simulink model "ModeloEstimacion"  (R2021a)
settings: Solver=ode4  StartTime=0.0  StopTime=10  FixedStep=0.005  MaxStep=1e-5  MinStep=1e-12  RelTol=1e-3
values from neighbouring files (symbols this model uses):
  A = theta(:,1:end-1)    [EstimacionLeon.m]
  B = (theta(:,end))    [EstimacionLeon.m]
undefined symbols (not defined in the file or in its folder): sigbuilder_block
settings Model: Creator=unam-  LastModifiedBy=jalej
settings DebuggingCC: UnconnectedInputMsg=none  UnconnectedOutputMsg=none  UnconnectedLineMsg=none
settings ModelReferenceCC: EnableRefExpFcnMdlSchedulingChecks=off
settings RTWCC: Description=Generic Real-Time Target  DLArmComputeVersion=20.02.1

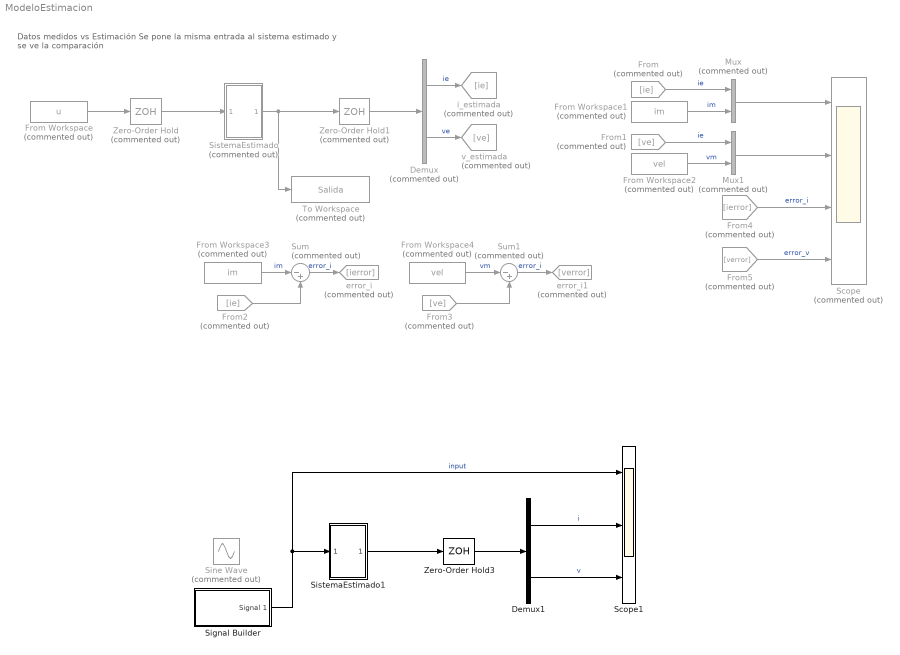
== system ModeloEstimacion ==
  note: Datos medidos vs Estimación
      | Se pone la misma entrada al sistema estimado y se ve la comparación
  Demux : Demux  Commented=on  Outputs=2
  Demux1 : Demux  Outputs=2
  From : From  Commented=on  GotoTag=ie
  From Workspace : FromWorkspace  Commented=on  VariableName=u  SampleTime=0.005
  From Workspace1 : FromWorkspace  Commented=on  VariableName=im
  From Workspace2 : FromWorkspace  Commented=on  VariableName=vel
  From Workspace3 : FromWorkspace  Commented=on  VariableName=im
  From Workspace4 : FromWorkspace  Commented=on  VariableName=vel
  From1 : From  Commented=on  GotoTag=ve
  From2 : From  Commented=on  GotoTag=ie
  From3 : From  Commented=on  GotoTag=ve
  From4 : From  Commented=on  GotoTag=ierror
  From5 : From  Commented=on  GotoTag=verror
  Mux : Mux  Commented=on  Inputs=2
  Mux1 : Mux  Commented=on  Inputs=2
  Scope : Scope  Commented=on  NumInputPorts=4
  Scope1 : Scope  NumInputPorts=3
  Signal Builder : Subsystem  Tag=STV Subsys  LoadFcn=sigbuilder_block('load');  StartFcn=sigbuilder_block('start');  StopFcn=sigbuilder_block('stop');  ClipboardFcn=sigbuilder_block('clipboard');  mask(Sigbuilder block){tuvar=[0:10]}
      mask help: Simulink:masks:SigbuilderBlock_MD
      mask init:
      | if ~strcmp(get_param(bdroot(gcbh),'SimulationStatus'),'stopped') tuvar = sigbuilder_block('maskInit'); end
      settings: CopyFcn=sigbuilder_block('copy');  DeleteFcn=sigbuilder_block('delete');  ModelCloseFcn=sigbuilder_block('modelClose');  PreSaveFcn=sigbuilder_block('preSave');  PauseFcn=sigbuilder_block('pause');  ContinueFcn=sigbuilder_block('continue');  NameChangeFcn=sigbuilder_block('namechange');  OpenFcn=sigbuilder_block('open',[437.6 199.2 550.4 400 ]);  CloseFcn=sigbuilder_block('close');
      mask Display: plot(0, 0, 100, 100,[2, 2, 32, 32, 2], [68, 8, 8, 68, 68],[32, 2], [38, 38], [32, 19, 2],[53, 60, 44], [32, 17, 17, 2],[16, 16, 31, 31]);txt = getActiveGroup(gcbh);text(2, 100, txt,'verticalAlignment', 'top');
  Sine Wave : Sin  Commented=on  Amplitude=6  Bias=6  SampleTime=0.005
  SistemaEstimado : Subsystem  Commented=on
  SistemaEstimado1 : Subsystem
  Sum : Sum  Commented=on  Inputs=|-+
  Sum1 : Sum  Commented=on  Inputs=|-+
  To Workspace : ToWorkspace  Commented=on  VariableName=Salida  SaveFormat=Timeseries  SampleTime=0.005
  Zero-Order Hold : ZeroOrderHold  Commented=on  SampleTime=0.005
  Zero-Order Hold1 : ZeroOrderHold  Commented=on  SampleTime=0.005
  Zero-Order Hold3 : ZeroOrderHold  SampleTime=0.005
  error_i : Goto  Commented=on  GotoTag=ierror
  error_i1 : Goto  Commented=on  GotoTag=verror
  i_estimada : Goto  Commented=on  GotoTag=ie
  v_estimada : Goto  Commented=on  GotoTag=ve
  wires:
  SistemaEstimado/1(Out1) -> To Workspace/1, Zero-Order Hold1/1
  Zero-Order Hold/1 -> SistemaEstimado/1(In1)
  Zero-Order Hold1/1 -> Demux/1
  From Workspace/1 -> Zero-Order Hold/1
  From Workspace2/1 -> Mux1/2  "vm"
  From Workspace1/1 -> Mux/2  "im"
  Mux/1 -> Scope/1
  Mux1/1 -> Scope/2
  Demux/1 -> i_estimada/1  "ie"
  Demux/2 -> v_estimada/1  "ve"
  From/1 -> Mux/1  "ie"
  From1/1 -> Mux1/1  "ie"
  From Workspace3/1 -> Sum/1  "im"
  From2/1 -> Sum/2
  Sum/1 -> error_i/1  "error_i"
  From Workspace4/1 -> Sum1/1  "vm"
  From3/1 -> Sum1/2
  Sum1/1 -> error_i1/1  "error_i"
  From4/1 -> Scope/3  "error_i"
  From5/1 -> Scope/4  "error_v"
  Demux1/2 -> Scope1/3  "v"
  SistemaEstimado1/1(Out1) -> Zero-Order Hold3/1
  Demux1/1 -> Scope1/2  "i"
  Zero-Order Hold3/1 -> Demux1/1
  Signal Builder/1(Signal 1) -> Scope1/1, SistemaEstimado1/1(In1)  "input"

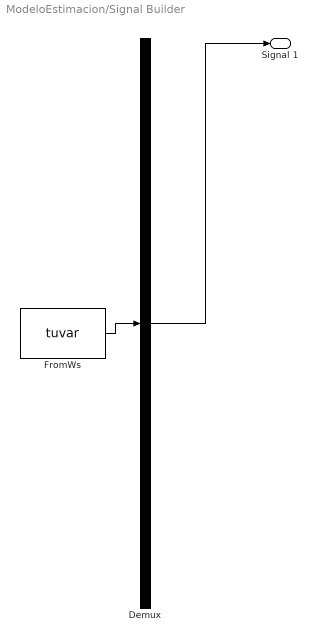
== system ModeloEstimacion/Signal Builder ==
  Demux : Demux  Tag=STV Demux  Outputs=1
      settings: DisplayOption=none
  FromWs : FromWorkspace  Tag=STV FromWs  VariableName=tuvar  SampleTime=0.005
      SigBuilderData=|
      | common.afterFinalStr = 'Extrapolate'
      | common.sampleTime = '0.005'
      | dataSet.timeRange = [0 10]
      | dataSet.name = 'Group 1'
      | sbobj.Groups.Name = 'Group 1'
      | sbobj.Groups.Signals.Name = 'Signal 1'
      | sbobj.Groups.Signals.XData = [0 2 2 9.02 9.02 10]
      | sbobj.Groups.Signals.YData = [0 0 12 12 0 0]
  Signal 1 : Outport  Tag=STV Outport
  wires:
  Demux/1 -> Signal 1/1
  FromWs/1 -> Demux/1

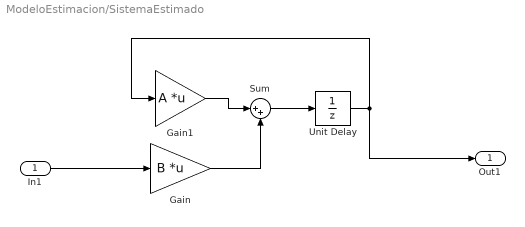
== system ModeloEstimacion/SistemaEstimado ==
  In1 : Inport
  Gain : Gain  Gain=B  Multiplication=Matrix(K*u)
  Gain1 : Gain  Gain=A  Multiplication=Matrix(K*u)
  Sum : Sum  Inputs=|++
  Unit Delay : UnitDelay  InitialCondition=[0.009670; 124.407227]  SampleTime=0.005  HasFrameUpgradeWarning=on
  Out1 : Outport
  wires:
  Unit Delay/1 -> Out1/1, Gain1/1
  Sum/1 -> Unit Delay/1
  Gain/1 -> Sum/2
  In1/1 -> Gain/1
  Gain1/1 -> Sum/1

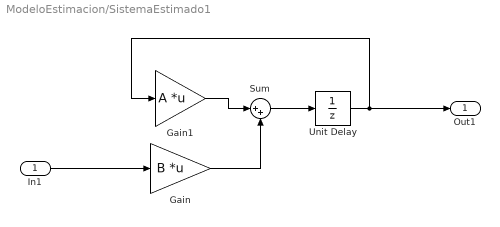
== system ModeloEstimacion/SistemaEstimado1 ==
  In1 : Inport
  Gain : Gain  Gain=B  Multiplication=Matrix(K*u)
  Gain1 : Gain  Gain=A  Multiplication=Matrix(K*u)
  Sum : Sum  Inputs=|++
  Unit Delay : UnitDelay  SampleTime=0.005  HasFrameUpgradeWarning=on
  Out1 : Outport
  wires:
  Unit Delay/1 -> Out1/1, Gain1/1
  Sum/1 -> Unit Delay/1
  Gain/1 -> Sum/2
  In1/1 -> Gain/1
  Gain1/1 -> Sum/1
